simulink model "script_model"  (R2023a)
settings: Solver=FixedStepAuto  StartTime=0.0  StopTime=10.0  FixedStep=ts  RelTol=1e-3
values from neighbouring files (symbols this model uses):
  Q = diag([0.1, 5, 0.1, 5])    [mpcdef.m]
  R = 1e-7    (= 1e-07)    [mpcdef.m]
  T_c = 6    [mpcdef.m]
  T_p = 12    [mpcdef.m]
  ts = 0.01    [mpcdef.m]
  u_lb = -2500    [mpcdef.m]
  u_ub = 2500    [mpcdef.m]
undefined symbols (not defined in the file or in its folder): A_d, B_d, C_d, D_d
libraries: simulink x1
settings Model: Creator=Adham  LastModifiedBy=Adham

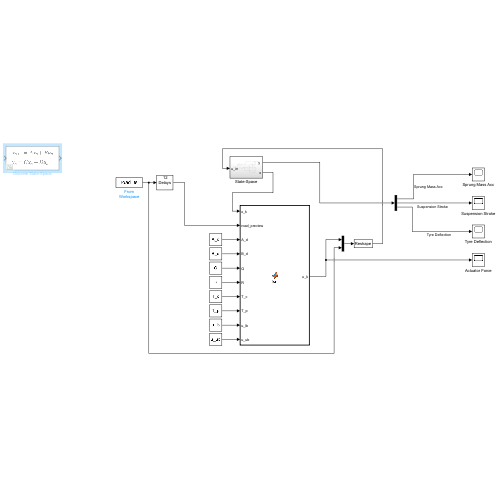
[thumbnail: Simulink's stored preview of the top-level diagram]
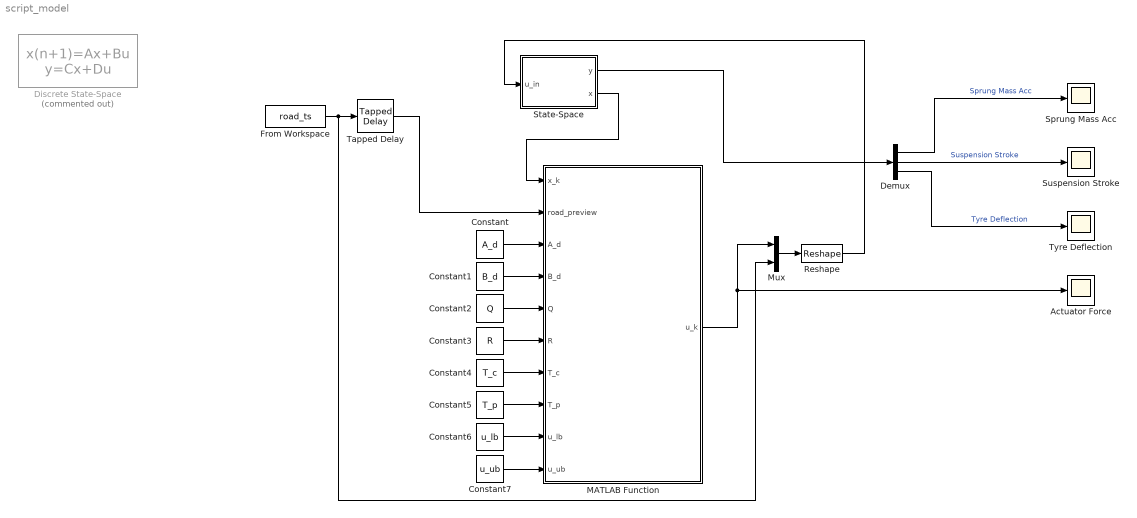
== system script_model ==
  Actuator Force : Scope
  Constant : Constant  Value=A_d
  Constant1 : Constant  Value=B_d
  Constant2 : Constant  Value=Q
  Constant3 : Constant  Value=R
  Constant4 : Constant  Value=T_c
  Constant5 : Constant  Value=T_p
  Constant6 : Constant  Value=u_lb
  Constant7 : Constant  Value=u_ub
  Demux : Demux  Outputs=3
  Discrete State-Space : DiscreteStateSpace  Commented=on  A=A_d  B=B_d  C=C_d  D=D_d  SampleTime=ts
  From Workspace : FromWorkspace  VariableName=road_ts
  MATLAB Function : MATLAB Function  TreatAsAtomicUnit=on
  Mux : Mux  Inputs=2
  Reshape : Reshape  OutputDimensionality=Customize  OutputDimensions=[2 1]
  Sprung Mass Acc : Scope
  State-Space : Subsystem
  Suspension Stroke : Scope
  Tapped Delay : simulink/Discrete/Tapped Delay  vinit=0.0  samptime=ts  NumDelays=T_p  DelayOrder=Oldest  includeCurrent=off
  Tyre Deflection : Scope
  wires:
  From Workspace/1 -> Tapped Delay/1, Mux/2
  Tapped Delay/1 -> MATLAB Function/2(road_preview)
  State-Space/2(x) -> MATLAB Function/1(x_k)
  MATLAB Function/1(u_k) -> Mux/1, Actuator Force/1
  Mux/1 -> Reshape/1
  Reshape/1 -> State-Space/1(u_in)
  Constant/1 -> MATLAB Function/3(A_d)
  Constant1/1 -> MATLAB Function/4(B_d)
  Constant2/1 -> MATLAB Function/5(Q)
  Constant3/1 -> MATLAB Function/6(R)
  Constant4/1 -> MATLAB Function/7(T_c)
  Constant5/1 -> MATLAB Function/8(T_p)
  Constant6/1 -> MATLAB Function/9(u_lb)
  Constant7/1 -> MATLAB Function/10(u_ub)
  State-Space/1("y ") -> Demux/1
  Demux/1 -> Sprung Mass Acc/1  "Sprung Mass Acc"
  Demux/2 -> Suspension Stroke/1  "Suspension Stroke"
  Demux/3 -> Tyre Deflection/1  "Tyre Deflection"

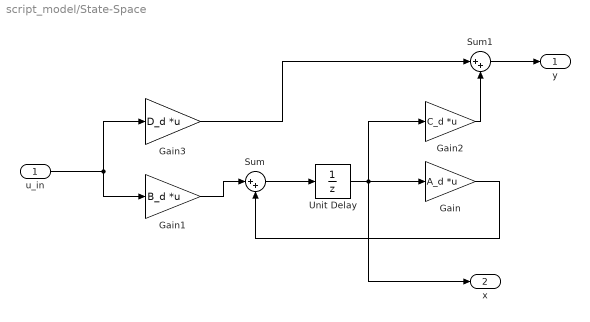
== system script_model/State-Space ==
  u_in : Inport
  Gain : Gain  Gain=A_d  Multiplication=Matrix(K*u)
  Gain1 : Gain  Gain=B_d  Multiplication=Matrix(K*u)
  Gain2 : Gain  Gain=C_d  Multiplication=Matrix(K*u)
  Gain3 : Gain  Gain=D_d  Multiplication=Matrix(K*u)
  Sum : Sum  Inputs=|++
  Sum1 : Sum  Inputs=|++
  Unit Delay : UnitDelay  InitialCondition=zeros(4,1)  SampleTime=ts  HasFrameUpgradeWarning=on
  "y " : Outport
  x : Outport  Port=2
  wires:
  Gain1/1 -> Sum/1
  Sum/1 -> Unit Delay/1
  Unit Delay/1 -> x/1, Gain/1, Gain2/1
  Gain3/1 -> Sum1/1
  Gain/1 -> Sum/2
  Sum1/1 -> "y "/1
  Gain2/1 -> Sum1/2
  u_in/1 -> Gain3/1, Gain1/1

== matlab function script_model/MATLAB Function ==
  data: x_k input; u_k output; road_preview input; A_d input; B_d input; Q input; R input; T_c input; T_p input; u_lb input; u_ub input
function u_k = fcn(x_k, road_preview, A_d, B_d, Q, R, T_c, T_p, u_lb, u_ub)
% This function implements the MPC logic for a single time step.
% All parameters are now passed as inputs.

% --- Optimization Problem Setup ---
u0 = zeros(T_c, 1); 
lb = repmat(u_lb, T_c, 1);
ub = repmat(u_ub, T_c, 1);

% Define the cost function to be minimized
cost_func = @(u) mpc_cost_function(u, A_d, B_d, Q, R, x_k, road_preview, T_c, T_p);

% Create a basic options structure for fmincon
options = optimoptions('fmincon','Display','none','Algorithm','sqp');

% Solve for the optimal control sequence using fmincon
u_optimal = fmincon(cost_func, u0, [], [], [], [], lb, ub, [], options);

% MPC rule: apply only the first element of the optimal sequence
u_k = u_optimal(1);

end


function cost = mpc_cost_function(u_seq, A_d, B_d, Q, R, x_0, z_road, T_c, T_p)
    cost = 0;
    x_k = x_0;
    
    for i = 1:T_c
        u_k = u_seq(i);
        dist_k = z_road(i);
        cost = cost + x_k'*Q*x_k + u_k'*R*u_k;
        x_k = A_d*x_k + B_d*[u_k; dist_k];
    end
    
    for i = T_c+1 : T_p
        dist_k = z_road(i);
        cost = cost + x_k'*Q*x_k;
        x_k = A_d*x_k + B_d*[0; dist_k];
    end
    cost = cost + x_k'*Q*x_k;
end
